simulink model "DCDC_BBC_hybrid1"  (R2020b)
settings: Solver=VariableStepAuto  StartTime=0.0  StopTime=10.0  RelTol=1e-3
values from neighbouring files (symbols this model uses):
  C_capacitance = 40e-3    (= 0.04)    [Hybrid1.m]    (also in Hybrid2.m; PID.m; PPO.m)
  error_threshold = 0.01    [Hybrid1.m]    (also in Hybrid2.m; PPO.m = 0.1)
  gain_K = 100    [Hybrid1.m]    (also in PID.m)
  init_action = 1    [Hybrid1.m]    (also in Hybrid2.m; PID.m; PPO.m)
  integral_I = 40000    [Hybrid1.m]    (also in PID.m)
  L_inductance = 10e-6    (= 1e-05)    [Hybrid1.m]    (also in Hybrid2.m; PID.m; PPO.m)
  periodVal = 1/10000    (= 0.0001)    [Hybrid1.m]    (also in PID.m)
  pw_percent = 50    [Hybrid1.m]    (also in PID.m)
  R_load = 100    [Hybrid1.m]    (also in Hybrid2.m; PID.m; PPO.m)
  stopping_criterion = 500    [Hybrid1.m]    (also in Hybrid2.m; PPO.m)
  V_ref = 30    [Hybrid1.m]    (also in Hybrid2.m; PID.m; PPO.m = 80)
  V_source_value = 48    [Hybrid1.m]    (also in Hybrid2.m; PID.m; PPO.m)
libraries: powerlib x8, rllib x1, pid_lib x1
settings Model: Creator=krupa  LastModifiedBy=krupa

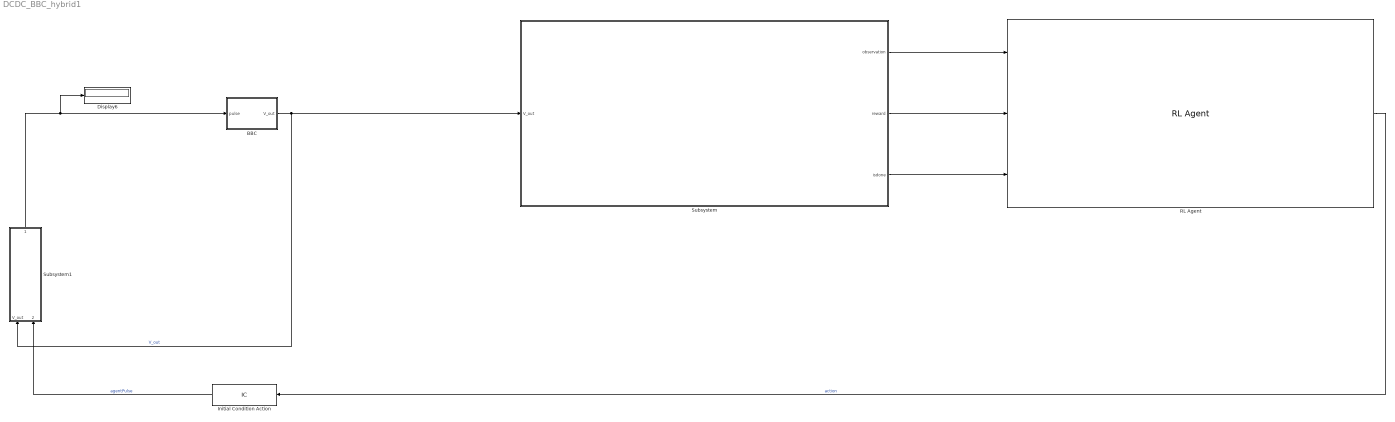
== system DCDC_BBC_hybrid1 ==
  BBC : Subsystem
  Display6 : Display
  Initial Condition Action : InitialCondition  Value=init_action
  RL Agent : rllib/RL Agent  Agent=agent  ProvideReward=on  ProvideIsDone=on  ProvideCumRwd=off  TreatAsDirectFeedthrough=on  CollectLoggedSignals=on  CollectModelStates=on
  Subsystem : Subsystem
  Subsystem1 : Subsystem
  wires:
  Subsystem/2(reward) -> RL Agent/2
  Subsystem/3(isdone) -> RL Agent/3
  Subsystem/1(observation) -> RL Agent/1
  RL Agent/1 -> Initial Condition Action/1  "action"
  BBC/1(V_out) -> Subsystem1/1(V_out), Subsystem/1(V_out)  "V_out"
  Subsystem1/1(action_applied) -> Display6/1, BBC/1(pulse)
  Initial Condition Action/1 -> Subsystem1/2(agentPulse)  "agentPulse"

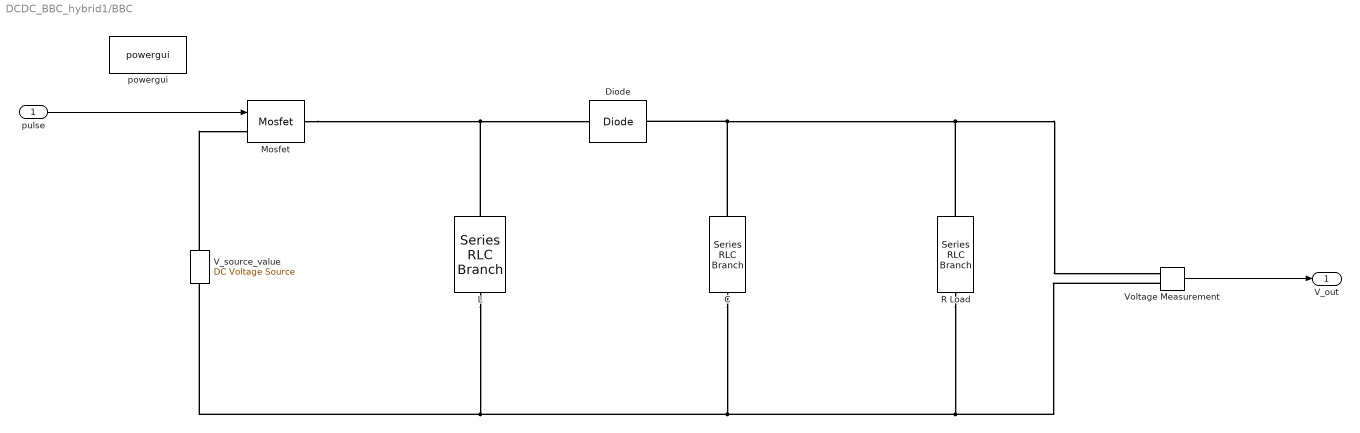
== system DCDC_BBC_hybrid1/BBC ==
  pulse : Inport
  C : powerlib/Elements/Series RLC Branch  LConnTagsString=__new0  RConnTagsString=__new0  BranchType=C  Resistance=1  Inductance=1e-3  SetiL0=off  InitialCurrent=0  Capacitance=C_capacitance  Setx0=off  InitialVoltage=0  Measurements=None
  Diode : powerlib/Power Electronics/Diode  Ron=0.001  Lon=0  Vf=0.8  IC=0  UseSnubber=0  Rs=500  Cs=250e-9  Measurements=off
  L : powerlib/Elements/Series RLC Branch  LConnTagsString=__new0  RConnTagsString=__new0  BranchType=L  Resistance=1  Inductance=L_inductance  SetiL0=off  InitialCurrent=0  Capacitance=1e-6  Setx0=off  InitialVoltage=0  Measurements=None
  Mosfet : powerlib/Power Electronics/Mosfet  Ron=0.1  Lon=0  Rd=0.01  Vfd=0  IC=0  Rs=1e5  Cs=inf  Measurements=off
  R Load : powerlib/Elements/Series RLC Branch  LConnTagsString=__new0  RConnTagsString=__new0  BranchType=R  Resistance=R_load  Inductance=1e-3  SetiL0=off  InitialCurrent=0  Capacitance=1e-6  Setx0=off  InitialVoltage=0  Measurements=None
  V_source_value : powerlib/Electrical Sources/DC Voltage Source  Amplitude=V_source_value  Measurements=None
  Voltage Measurement : powerlib/Measurements/Voltage Measurement  PhasorSimulation=off  OutputType=Complex  PSBequivalent=0
  powergui : powerlib/powergui  Priority=1  SimulationMode=Continuous  SampleTime=50e-6  frequency=60  Iterations=50  frequencyindice=0  Pbase=100e6  ErrMax=1e-4  UnitsV=kV  UnitsW=MW  buscounter=0  FunctionMessages=off  echomessages=off  EnableUseOfTLC=off  CurrentSourceSwitches=off  DisableSnubberDevices=off  DisableRonSwitches=off  DisableVfSwitches=off  DisplayEquations=off  AutomaticDiscreteSolvers=off  SolverType=Tustin/Backward Euler (TBE)  Interpol=off  ExternalGateDelay=off  methode=off  Ts=100  x0status=blocks  SPID=on  SwTol=0  HookPort=off  NonlinearTolerance=1e-4  nMaxIteration=100  ContinueOnMaxIteration=off  RestoreLinks=warning  ResistiveCurrentMeasurement=off  Frange=[0:2:500]  Ylog=off  Xlog=on  ShowGrid=off  save=off  variable=ZData  structure=0  ZoomFFT=off  StartTime=0.0  cycles=1  DisplayStyle=1  fundamental=60  FreqAxis=off  MaxFrequency=1000  frequencyindicesteady=1  RmsSteady=1  display=off
  V_out : Outport
  wires:
  Voltage Measurement/1 -> V_out/1
  pulse/1 -> Mosfet/1
  connections:
  V_source_value/RConn1 -- Mosfet/LConn1
  C/RConn1 -- Voltage Measurement/LConn1 -- R Load/RConn1 -- Diode/LConn1
  L/RConn1 -- Diode/RConn1 -- Mosfet/RConn1
  R Load/LConn1 -- Voltage Measurement/LConn2 -- C/LConn1 -- L/LConn1 -- V_source_value/LConn1

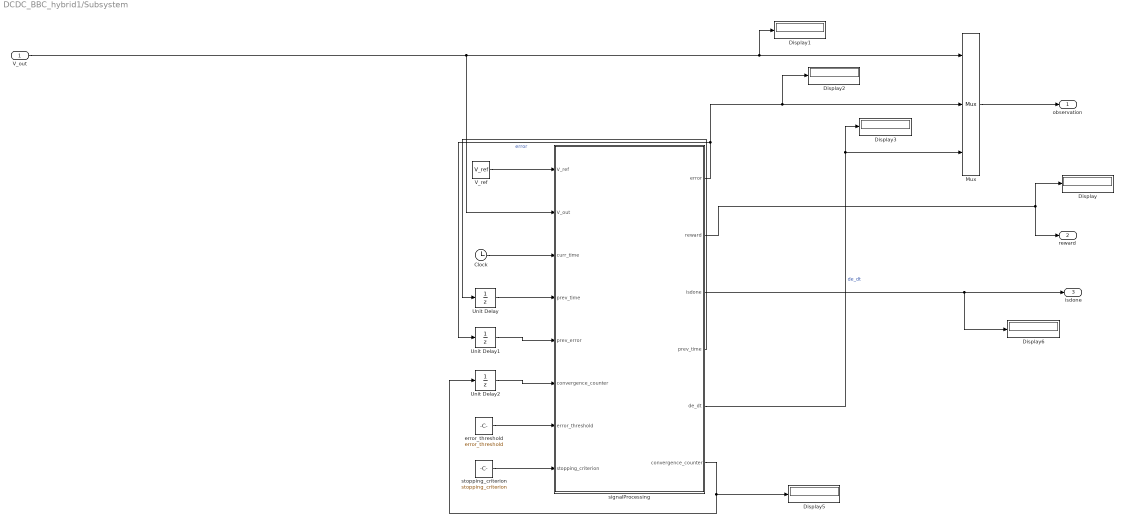
== system DCDC_BBC_hybrid1/Subsystem ==
  V_out : Inport
  Clock : Clock
  Display{,1..3,5..6} (6 alike) : Display
  Mux : Mux  Inputs=3
  Unit Delay : UnitDelay  SampleTime=-1  HasFrameUpgradeWarning=on
  Unit Delay1 : UnitDelay  SampleTime=-1  HasFrameUpgradeWarning=on
  Unit Delay2 : UnitDelay  SampleTime=-1  HasFrameUpgradeWarning=on
  V_ref : Constant  Value=V_ref
  error_threshold : Constant  Value=error_threshold
  signalProcessing : MATLAB Function  TreatAsAtomicUnit=on
  stopping_criterion : Constant  Value=stopping_criterion
  observation : Outport
  reward : Outport  Port=2
  isdone : Outport  Port=3
  wires:
  V_out/1 -> signalProcessing/2(V_out), Display1/1, Mux/1
  Unit Delay/1 -> signalProcessing/4("prev_time ")
  signalProcessing/2(reward) -> reward/1, Display/1
  V_ref/1 -> signalProcessing/1(V_ref)
  Mux/1 -> observation/1
  Unit Delay2/1 -> signalProcessing/6("convergence_counter ")
  signalProcessing/3(isdone) -> Display6/1, isdone/1
  Unit Delay1/1 -> signalProcessing/5(prev_error)
  signalProcessing/6(convergence_counter) -> Display5/1, Unit Delay2/1
  signalProcessing/1(error) -> Unit Delay1/1, Display2/1, Mux/2  "error"
  signalProcessing/5(de_dt) -> Display3/1, Mux/3  "de_dt"
  Clock/1 -> signalProcessing/3(curr_time)
  error_threshold/1 -> signalProcessing/7(error_threshold)
  stopping_criterion/1 -> signalProcessing/8(stopping_criterion)
  signalProcessing/4(prev_time) -> Unit Delay/1

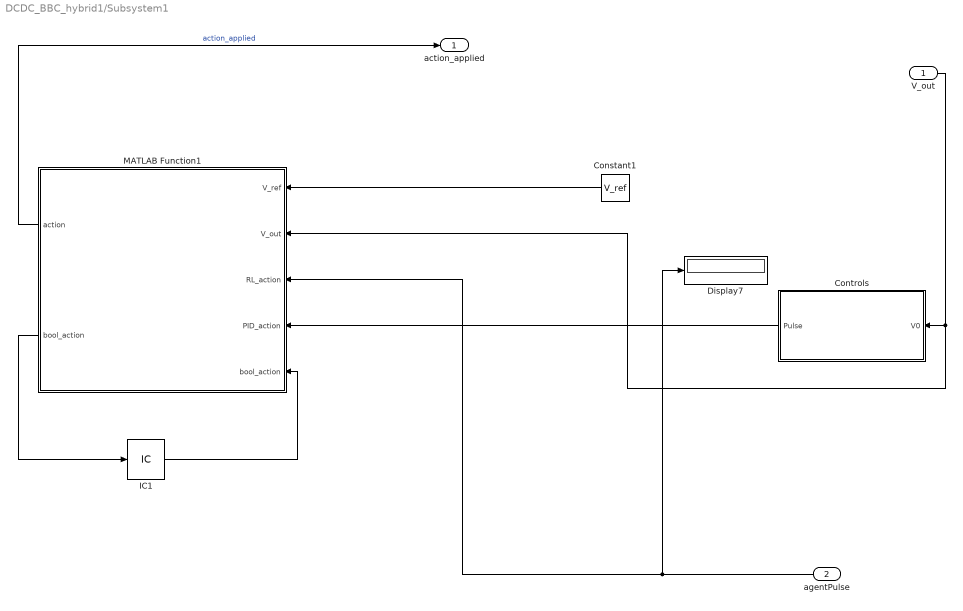
== system DCDC_BBC_hybrid1/Subsystem1 ==
  V_out : Inport
  agentPulse : Inport  Port=2
  Constant1 : Constant  Value=V_ref
  Controls : Subsystem
  Display7 : Display
  IC1 : InitialCondition  Value=0
  MATLAB Function1 : MATLAB Function  TreatAsAtomicUnit=on
  action_applied : Outport
  wires:
  agentPulse/1 -> Display7/1, MATLAB Function1/3(RL_action)
  V_out/1 -> MATLAB Function1/2(V_out), Controls/1(V0)
  Controls/1(Pulse) -> MATLAB Function1/4(PID_action)
  IC1/1 -> MATLAB Function1/5("bool_action ")
  Constant1/1 -> MATLAB Function1/1(V_ref)
  MATLAB Function1/1(action) -> action_applied/1  "action_applied"
  MATLAB Function1/2(bool_action) -> IC1/1

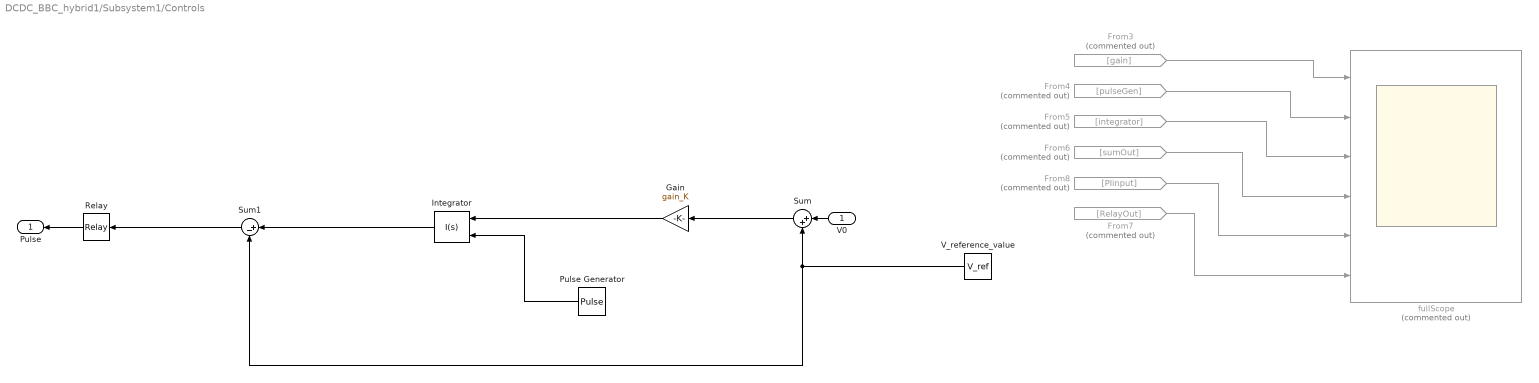
== system DCDC_BBC_hybrid1/Subsystem1/Controls ==
  V0 : Inport
  From3 : From  Commented=on  GotoTag=gain
  From4 : From  Commented=on  GotoTag=pulseGen
  From5 : From  Commented=on  GotoTag=integrator
  From6 : From  Commented=on  GotoTag=sumOut
  From7 : From  Commented=on  GotoTag=RelayOut
  From8 : From  Commented=on  GotoTag=PIinput
  Gain : Gain  Gain=gain_K
  Integrator : pid_lib/PID Controller  Controller=I  Form=Parallel  TimeDomain=Continuous-time  UseExternalTs=off  SampleTime=-1  IntegratorMethod=Forward Euler  FilterMethod=Forward Euler  ControllerParametersSource=internal  P=1  I=integral_I  D=0  UseFilter=on  N=100  TunerSelectOption=Transfer Function Based (PID Tuner App)  InitialConditionSource=internal  InitialConditionForIntegrator=0  InitialConditionForFilter=0  DifferentiatorICPrevScaledInput=0  ExternalReset=rising  TrackingMode=off  Kt=1  LimitOutput=off  SatLimitsSource=internal  UpperSaturationLimit=inf  LowerSaturationLimit=-inf  LinearizeAsGain=off  AntiWindupMode=none  Kb=1  POutMin=[]  POutMax=[]  IOutMin=[]  IOutMax=[]  DOutMin=[]  DOutMax=[]  NOutMin=[]  NOutMax=[]  SumOutMin=[]  SumOutMax=[]  SaturationOutMin=[]  SaturationOutMax=[]  PParamMin=[]  PParamMax=[]  IParamMin=[]  IParamMax=[]  DParamMin=[]  DParamMax=[]  NParamMin=[]  NParamMax=[]  KbParamMin=[]  KbParamMax=[]  KtParamMin=[]  KtParamMax=[]  KbOutMin=[]  KbOutMax=[]  KtOutMin=[]  KtOutMax=[]  IntegratorOutMin=[]  IntegratorOutMax=[]  FilterOutMin=[]  FilterOutMax=[]  SumI1OutMin=[]  SumI1OutMax=[]  SumI2OutMin=[]  SumI2OutMax=[]  SumI3OutMin=[]  SumI3OutMax=[]  SumI4OutMin=[]  SumI4OutMax=[]  SumDOutMin=[]  SumDOutMax=[]  DifferentiatorOutMin=[]  DifferentiatorOutMax=[]  FilterDiffOutCoefMin=[]  FilterDiffOutCoefMax=[]  ReciprocalOutMin=[]  ReciprocalOutMax=[]  SumDenOutMin=[]  SumDenOutMax=[]  SumNumOutMin=[]  SumNumOutMax=[]  DivideOutMin=[]  DivideOutMax=[]  UdiffTsProdOutMin=[]  UdiffTsProdOutMax=[]  NTsProdOutMin=[]  NTsProdOutMax=[]  UintegralTsProdOutMin=[]  UintegralTsProdOutMax=[]  UngainTsProdOutMin=[]  UngainTsProdOutMax=[]  IntegratorContinuousStateAttributes=''  IntegratorStateMustResolveToSignalObject=off  IntegratorRTWStateStorageClass=Auto  FilterContinuousStateAttributes=''  FilterStateMustResolveToSignalObject=off  FilterRTWStateStorageClass=Auto  ParallelPVariant=Disabled  IdealPVariant=Disabled  IVariant=InternalParameters  DVariant=Disabled  IntegratorVariant=Continuous  SatVariant=Disabled  AWVariant=Passthrough  PCopyVariant=Disabled  TRVariant=Disabled  FdbkBlocksVariant=Forward  IdealPFdbkVariant=Disabled  SatFdbkVariant=Disabled  DerivativeFilterVariant=Disabled  NVariant=Disabled  NCopyVariant=Disabled_SignalSpec  FilterICVariant=Disabled  IntegratorICVariant=InternalICs  ExternalResetVariant=ExternalReset  TRSumVariant=Passthrough  SumFdbkVariant=Disabled  SumVariant=Passthrough_I  TsampFilterVariant=InternalTs  TsampNgainVariant=Passthrough  TsampIntegralVariant=Passthrough  ExternalSaturationOutDataTypeStr=Inherit: Same as second input
  Pulse Generator : DiscretePulseGenerator  PulseType=Time based  Period=periodVal  PulseWidth=pw_percent
  Relay : Relay
  Sum : Sum  Inputs=|++
  Sum1 : Sum  Inputs=|+-
  V_reference_value : Constant  Value=V_ref
  fullScope : Scope  Commented=on  NumInputPorts=6
  Pulse : Outport
  wires:
  Sum/1 -> Gain/1
  V0/1 -> Sum/1
  Gain/1 -> Integrator/1
  Relay/1 -> Pulse/1
  Sum1/1 -> Relay/1
  Integrator/1 -> Sum1/1
  V_reference_value/1 -> Sum1/2, Sum/2
  Pulse Generator/1 -> Integrator/2
  From8/1 -> fullScope/5
  From4/1 -> fullScope/2
  From3/1 -> fullScope/1
  From7/1 -> fullScope/6
  From6/1 -> fullScope/4
  From5/1 -> fullScope/3

== matlab function DCDC_BBC_hybrid1/Subsystem1/MATLAB Function1 ==
  data: V_ref input; V_out input; action output; RL_action input; PID_action input; bool_action input; bool_action output
function [action, bool_action] = fcn(V_ref, V_out, RL_action, PID_action, bool_action)
if bool_action == 1
    action = PID_action;
else
    if abs(V_out)>=V_ref
        action= PID_action;
        bool_action = 1;
    else
        action = RL_action;
    end
end

== matlab function DCDC_BBC_hybrid1/Subsystem/signalProcessing ==
  data: V_ref input; error output; V_out input; curr_time input; prev_time input; prev_error input; convergence_counter input; error_threshold input; stopping_criterion input; reward output; isdone output; prev_time output; de_dt output; convergence_counter output
function [error, reward, isdone, prev_time, de_dt, convergence_counter] = signalProcessing(V_ref, V_out, curr_time, prev_time, prev_error, convergence_counter, error_threshold, stopping_criterion)
%error
abs_Vout = abs(V_out);
error = V_ref - abs_Vout;
abs_error = abs(error);

% change in error
de_dt = (prev_error - error)/(curr_time - prev_time);

isdone = 0;
prev_time = curr_time; 

% convergence criterion
if abs_error <= error_threshold
    convergence_counter = convergence_counter +1;
    if convergence_counter >= stopping_criterion
        isdone = 1;
    end
else
    convergence_counter = 0;
end


if abs_Vout<=(V_ref+error_threshold)
    if abs_error<abs(prev_error)
        reward = 1/abs_error;
    else
        reward = -1/abs_error;
    end
else
    reward = -abs_error;
end
% reward = 1/abs_error;




% if abs_Vout <= (V_ref+error_threshold)
%     if abs_error<=abs(prev_error)
%         reward = 1/abs_error;
%     else
%         reward = -1/abs_error;
%     end
% else
%     reward = -abs_error;
% end

% if abs_Vout == V_ref
%     reward = 100;
% elseif abs_Vout<V_ref
%    reward = (0.25*(1-(curr_time/Tf))) + (0.5*(V_out/V_ref)) + (0.25*(1-(error/prev_error)));
% elseif abs_Vout <= (V_ref+error_threshold)
%     reward = 
% end
